simulink model "parallelForm"  (R2024a)
settings: Solver=VariableStepAuto  StartTime=0.0  StopTime=10.0  RelTol=1e-3
settings Model: Creator=prath  LastModifiedBy=prath

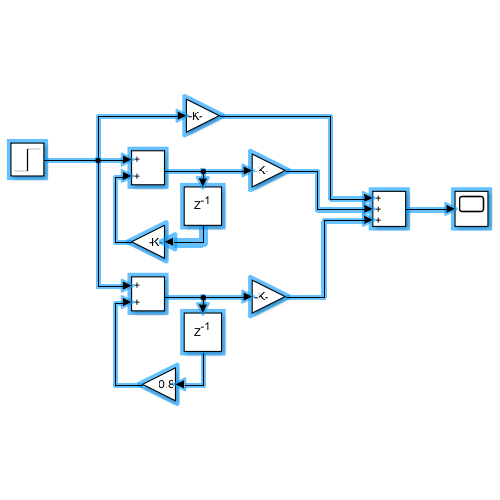
[thumbnail: Simulink's stored preview of the top-level diagram]
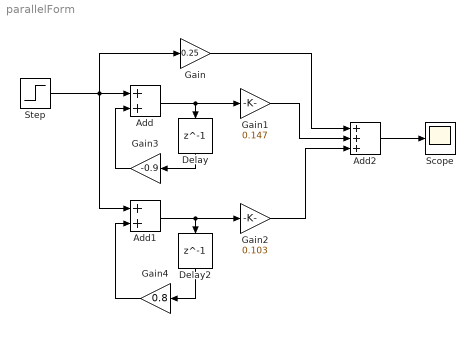
== system parallelForm ==
  Add : Sum
  Add1 : Sum
  Add2 : Sum  Inputs=+++
  Delay : Delay  DelayLength=1
  Delay2 : Delay  DelayLength=1
  Gain : Gain  Gain=0.25
  Gain1 : Gain  Gain=0.147
  Gain2 : Gain  Gain=0.103
  Gain3 : Gain  Gain=-0.9
  Gain4 : Gain  Gain=0.8
  Scope : Scope
  Step : Step  SampleTime=0
  wires:
  Add2/1 -> Scope/1
  Gain1/1 -> Add2/2
  Gain4/1 -> Add1/2
  Delay2/1 -> Gain4/1
  Add/1 -> Gain1/1, Delay/1
  Gain2/1 -> Add2/3
  Gain3/1 -> Add/2
  Add1/1 -> Gain2/1, Delay2/1
  Gain/1 -> Add2/1
  Step/1 -> Add1/1, Gain/1, Add/1
  Delay/1 -> Gain3/1
